simulink model "firefliesDemo"  (Simulink 7.4)
settings: Solver=ode3  StartTime=0.0  StopTime=200  FixedStep=1  RelTol=1e-3
values from neighbouring files (symbols this model uses):
  K = 2.5    [firefliesDemo.mat]
  N = 5    [clusterDemo.mat]    (also in firefliesDemo.mat = 10)
  omega = 0.628318530718    [firefliesDemo.mat]
  rho0 = 10    [firefliesDemo.mat]
  threshold = 0.8    [firefliesDemo.mat]
  var = 0    [clusterDemo.mat]    (also in firefliesDemo.mat = 3)
(part 2 of 2)

== system firefliesDemo/Node8 ==
  In1 : Inport  OutDataType=fixdt(1, 16)  OutScaling=2^0
  In2 : Inport  Port=2
  In3 : Inport  Port=3
  In4 : Inport  Port=4
  In5 : Inport  Port=5
  In6 : Inport  Port=6
  In7 : Inport  Port=7
  In8 : Inport  Port=8
  In10 : Inport  Port=9
  In11 : Inport  Port=10
  In12 : Inport  Port=11
  In13 : Inport  Port=12
  In14 : Inport  Port=13
  In15 : Inport  Port=14
  In16 : Inport  Port=15
  In17 : Inport  Port=16
  In18 : Inport  Port=17
  In19 : Inport  Port=18
  In20 : Inport  Port=19
  Add : Sum  OutDataType=fixdt(1, 16)  OutScaling=2^-10
  Add1 : Sum  Inputs=+-  OutDataType=fixdt(1, 16)  OutScaling=2^-10
  Gain : Gain  Gain=K/N  ParameterDataType=fixdt(1, 16)  ParameterScaling=2^0  OutDataType=fixdt(1, 16)  OutScaling=2^0
  Integrator : Integrator  InitialConditionSource=external
  Math Function : Math  Operator=mod  OutDataType=fixdt(1, 16)  OutScaling=2^0  SaturateOnIntegerOverflow=on
  Mux : Mux  Inputs=19
  Scope : Scope
  Scope2 : Scope
      settings: SaveName=ScopeData2
  Sum of Elements : Sum  Inputs=+  OutDataType=fixdt(1, 16)  OutScaling=2^-10
  Threshold : Constant  Value=threshold  OutDataType=fixdt(1, 16)  OutScaling=2^0
  Trigonometric Function : Trigonometry
  angle speed : Constant  Value=omega  OutDataType=fixdt(1, 16)  OutScaling=2^0
  flash : Stateflow chart
  period : Constant  Value=2*pi  OutDataType=fixdt(1, 16)  OutScaling=2^0
  rho0 : Constant  Value=rho0+rand(1)*var  OutDataType=fixdt(1, 16)  OutScaling=2^0
  Out1 : Outport  OutDataType=fixdt(1, 16)  OutScaling=2^0
  wires:
  In20/1 -> Mux/19
  In19/1 -> Mux/18
  In18/1 -> Mux/17
  In17/1 -> Mux/16
  In16/1 -> Mux/15
  In15/1 -> Mux/14
  In14/1 -> Mux/13
  In13/1 -> Mux/12
  In12/1 -> Mux/11
  In11/1 -> Mux/10
  In10/1 -> Mux/9
  In8/1 -> Mux/8
  In7/1 -> Mux/7
  In6/1 -> Mux/6
  In5/1 -> Mux/5
  In4/1 -> Mux/4
  In3/1 -> Mux/3
  In2/1 -> Mux/2
  Threshold/1 -> flash/2(t)
  Math Function/1 -> flash/1(u), Scope2/1
  period/1 -> Math Function/2
  rho0/1 -> Integrator/2
  Sum of Elements/1 -> Gain/1
  Trigonometric Function/1 -> Sum of Elements/1
  Add/1 -> Integrator/1  "drho/dt"
  Gain/1 -> Add/2
  angle speed/1 -> Add/1
  Add1/1 -> Trigonometric Function/1
  Integrator/1 -> Math Function/1, Scope/1, Out1/1, Add1/2  "rho_i"
  Mux/1 -> Add1/1
  In1/1 -> Mux/1

== system firefliesDemo/Node9 ==
  In1 : Inport  OutDataType=fixdt(1, 16)  OutScaling=2^0
  In2 : Inport  Port=2
  In3 : Inport  Port=3
  In4 : Inport  Port=4
  In5 : Inport  Port=5
  In6 : Inport  Port=6
  In7 : Inport  Port=7
  In8 : Inport  Port=8
  In9 : Inport  Port=9
  In11 : Inport  Port=10
  In12 : Inport  Port=11
  In13 : Inport  Port=12
  In14 : Inport  Port=13
  In15 : Inport  Port=14
  In16 : Inport  Port=15
  In17 : Inport  Port=16
  In18 : Inport  Port=17
  In19 : Inport  Port=18
  In20 : Inport  Port=19
  Add : Sum  OutDataType=fixdt(1, 16)  OutScaling=2^-10
  Add1 : Sum  Inputs=+-  OutDataType=fixdt(1, 16)  OutScaling=2^-10
  Gain : Gain  Gain=K/N  ParameterDataType=fixdt(1, 16)  ParameterScaling=2^0  OutDataType=fixdt(1, 16)  OutScaling=2^0
  Integrator : Integrator  InitialConditionSource=external
  Math Function : Math  Operator=mod  OutDataType=fixdt(1, 16)  OutScaling=2^0  SaturateOnIntegerOverflow=on
  Mux : Mux  Inputs=19
  Scope : Scope
  Scope2 : Scope
      settings: SaveName=ScopeData2
  Sum of Elements : Sum  Inputs=+  OutDataType=fixdt(1, 16)  OutScaling=2^-10
  Threshold : Constant  Value=threshold  OutDataType=fixdt(1, 16)  OutScaling=2^0
  Trigonometric Function : Trigonometry
  angle speed : Constant  Value=omega  OutDataType=fixdt(1, 16)  OutScaling=2^0
  flash : Stateflow chart
  period : Constant  Value=2*pi  OutDataType=fixdt(1, 16)  OutScaling=2^0
  rho0 : Constant  Value=rho0+rand(1)*var  OutDataType=fixdt(1, 16)  OutScaling=2^0
  Out1 : Outport  OutDataType=fixdt(1, 16)  OutScaling=2^0
  wires:
  In20/1 -> Mux/19
  In19/1 -> Mux/18
  In18/1 -> Mux/17
  In17/1 -> Mux/16
  In16/1 -> Mux/15
  In15/1 -> Mux/14
  In14/1 -> Mux/13
  In13/1 -> Mux/12
  In12/1 -> Mux/11
  In11/1 -> Mux/10
  In9/1 -> Mux/9
  In8/1 -> Mux/8
  In7/1 -> Mux/7
  In6/1 -> Mux/6
  In5/1 -> Mux/5
  In4/1 -> Mux/4
  In3/1 -> Mux/3
  In2/1 -> Mux/2
  Threshold/1 -> flash/2(t)
  Math Function/1 -> flash/1(u), Scope2/1
  period/1 -> Math Function/2
  rho0/1 -> Integrator/2
  Sum of Elements/1 -> Gain/1
  Trigonometric Function/1 -> Sum of Elements/1
  Add/1 -> Integrator/1  "drho/dt"
  Gain/1 -> Add/2
  angle speed/1 -> Add/1
  Add1/1 -> Trigonometric Function/1
  Integrator/1 -> Math Function/1, Scope/1, Out1/1, Add1/2  "rho_i"
  Mux/1 -> Add1/1
  In1/1 -> Mux/1

== matlab function Node1/flash ==
  data: u input double; y output double; t input double
function y = fcn(u,t)
%#eml
% Allows the flashing of the subsystem block after some threshold
eml.extrinsic('set_param','get_param','gcs');

y = u;

if u > t
set_param(get_param(gcs,'parent'),'BackgroundColor','[0.3, 0.9, 0.5]');
else
set_param(get_param(gcs,'parent'),'BackgroundColor','black');
end

y = u;

== matlab function Node/flash ==
  data: u input double; y output double; t input double
function y = fcn(u,t)
%#eml
% Allows the flashing of the subsystem block after some threshold
eml.extrinsic('set_param','get_param','gcs');

y = u;

if u > t
set_param(get_param(gcs,'parent'),'BackgroundColor','[0.3, 0.9, 0.5]');
else
set_param(get_param(gcs,'parent'),'BackgroundColor','black');
end

y = u;

== matlab function Node2/flash ==
  data: u input double; y output double; t input double
function y = fcn(u,t)
%#eml
% Allows the flashing of the subsystem block after some threshold
eml.extrinsic('set_param','get_param','gcs');

y = u;

if u > t
set_param(get_param(gcs,'parent'),'BackgroundColor','[0.3, 0.9, 0.5]');
else
set_param(get_param(gcs,'parent'),'BackgroundColor','black');
end

y = u;

== matlab function Node3/flash ==
  data: u input double; y output double; t input double
function y = fcn(u,t)
%#eml
% Allows the flashing of the subsystem block after some threshold
eml.extrinsic('set_param','get_param','gcs');

y = u;

if u > t
set_param(get_param(gcs,'parent'),'BackgroundColor','[0.3, 0.9, 0.5]');
else
set_param(get_param(gcs,'parent'),'BackgroundColor','black');
end

y = u;

== matlab function Node4/flash ==
  data: u input double; y output double; t input double
function y = fcn(u,t)
%#eml
% Allows the flashing of the subsystem block after some threshold
eml.extrinsic('set_param','get_param','gcs');

y = u;

if u > t
set_param(get_param(gcs,'parent'),'BackgroundColor','[0.3, 0.9, 0.5]');
else
set_param(get_param(gcs,'parent'),'BackgroundColor','black');
end

y = u;

== matlab function Node5/flash ==
  data: u input double; y output double; t input double
function y = fcn(u,t)
%#eml
% Allows the flashing of the subsystem block after some threshold
eml.extrinsic('set_param','get_param','gcs');

y = u;

if u > t
set_param(get_param(gcs,'parent'),'BackgroundColor','[0.3, 0.9, 0.5]');
else
set_param(get_param(gcs,'parent'),'BackgroundColor','black');
end

y = u;

== matlab function Node6/flash ==
  data: u input double; y output double; t input double
function y = fcn(u,t)
%#eml
% Allows the flashing of the subsystem block after some threshold
eml.extrinsic('set_param','get_param','gcs');

y = u;

if u > t
set_param(get_param(gcs,'parent'),'BackgroundColor','[0.3, 0.9, 0.5]');
else
set_param(get_param(gcs,'parent'),'BackgroundColor','black');
end

y = u;

== matlab function Node7/flash ==
  data: u input double; y output double; t input double
function y = fcn(u,t)
%#eml
% Allows the flashing of the subsystem block after some threshold
eml.extrinsic('set_param','get_param','gcs');

y = u;

if u > t
set_param(get_param(gcs,'parent'),'BackgroundColor','[0.3, 0.9, 0.5]');
else
set_param(get_param(gcs,'parent'),'BackgroundColor','black');
end

y = u;

== matlab function Node8/flash ==
  data: u input double; y output double; t input double
function y = fcn(u,t)
%#eml
% Allows the flashing of the subsystem block after some threshold
eml.extrinsic('set_param','get_param','gcs');

y = u;

if u > t
set_param(get_param(gcs,'parent'),'BackgroundColor','[0.3, 0.9, 0.5]');
else
set_param(get_param(gcs,'parent'),'BackgroundColor','black');
end

y = u;

== matlab function Node9/flash ==
  data: u input double; y output double; t input double
function y = fcn(u,t)
%#eml
% Allows the flashing of the subsystem block after some threshold
eml.extrinsic('set_param','get_param','gcs');

y = u;

if u > t
set_param(get_param(gcs,'parent'),'BackgroundColor','[0.3, 0.9, 0.5]');
else
set_param(get_param(gcs,'parent'),'BackgroundColor','black');
end

y = u;

== matlab function Node10/flash ==
  data: u input double; y output double; t input double
function y = fcn(u,t)
%#eml
% Allows the flashing of the subsystem block after some threshold
eml.extrinsic('set_param','get_param','gcs');

y = u;

if u > t
set_param(get_param(gcs,'parent'),'BackgroundColor','[0.3, 0.9, 0.5]');
else
set_param(get_param(gcs,'parent'),'BackgroundColor','black');
end

y = u;

== matlab function Node11/flash ==
  data: u input double; y output double; t input double
function y = fcn(u,t)
%#eml
% Allows the flashing of the subsystem block after some threshold
eml.extrinsic('set_param','get_param','gcs');

y = u;

if u > t
set_param(get_param(gcs,'parent'),'BackgroundColor','[0.3, 0.9, 0.5]');
else
set_param(get_param(gcs,'parent'),'BackgroundColor','black');
end

y = u;

== matlab function Node12/flash ==
  data: u input double; y output double; t input double
function y = fcn(u,t)
%#eml
% Allows the flashing of the subsystem block after some threshold
eml.extrinsic('set_param','get_param','gcs');

y = u;

if u > t
set_param(get_param(gcs,'parent'),'BackgroundColor','[0.3, 0.9, 0.5]');
else
set_param(get_param(gcs,'parent'),'BackgroundColor','black');
end

y = u;

== matlab function Node13/flash ==
  data: u input double; y output double; t input double
function y = fcn(u,t)
%#eml
% Allows the flashing of the subsystem block after some threshold
eml.extrinsic('set_param','get_param','gcs');

y = u;

if u > t
set_param(get_param(gcs,'parent'),'BackgroundColor','[0.3, 0.9, 0.5]');
else
set_param(get_param(gcs,'parent'),'BackgroundColor','black');
end

y = u;

== matlab function Node14/flash ==
  data: u input double; y output double; t input double
function y = fcn(u,t)
%#eml
% Allows the flashing of the subsystem block after some threshold
eml.extrinsic('set_param','get_param','gcs');

y = u;

if u > t
set_param(get_param(gcs,'parent'),'BackgroundColor','[0.3, 0.9, 0.5]');
else
set_param(get_param(gcs,'parent'),'BackgroundColor','black');
end

y = u;

== matlab function Node15/flash ==
  data: u input double; y output double; t input double
function y = fcn(u,t)
%#eml
% Allows the flashing of the subsystem block after some threshold
eml.extrinsic('set_param','get_param','gcs');

y = u;

if u > t
set_param(get_param(gcs,'parent'),'BackgroundColor','[0.3, 0.9, 0.5]');
else
set_param(get_param(gcs,'parent'),'BackgroundColor','black');
end

y = u;

== matlab function Node16/flash ==
  data: u input double; y output double; t input double
function y = fcn(u,t)
%#eml
% Allows the flashing of the subsystem block after some threshold
eml.extrinsic('set_param','get_param','gcs');

y = u;

if u > t
set_param(get_param(gcs,'parent'),'BackgroundColor','[0.3, 0.9, 0.5]');
else
set_param(get_param(gcs,'parent'),'BackgroundColor','black');
end

y = u;

== matlab function Node17/flash ==
  data: u input double; y output double; t input double
function y = fcn(u,t)
%#eml
% Allows the flashing of the subsystem block after some threshold
eml.extrinsic('set_param','get_param','gcs');

y = u;

if u > t
set_param(get_param(gcs,'parent'),'BackgroundColor','[0.3, 0.9, 0.5]');
else
set_param(get_param(gcs,'parent'),'BackgroundColor','black');
end

y = u;

== matlab function Node18/flash ==
  data: u input double; y output double; t input double
function y = fcn(u,t)
%#eml
% Allows the flashing of the subsystem block after some threshold
eml.extrinsic('set_param','get_param','gcs');

y = u;

if u > t
set_param(get_param(gcs,'parent'),'BackgroundColor','[0.3, 0.9, 0.5]');
else
set_param(get_param(gcs,'parent'),'BackgroundColor','black');
end

y = u;

== matlab function Node19/flash ==
  data: u input double; y output double; t input double
function y = fcn(u,t)
%#eml
% Allows the flashing of the subsystem block after some threshold
eml.extrinsic('set_param','get_param','gcs');

y = u;

if u > t
set_param(get_param(gcs,'parent'),'BackgroundColor','[0.3, 0.9, 0.5]');
else
set_param(get_param(gcs,'parent'),'BackgroundColor','black');
end

y = u;
